simulink model "EKF"  (R2021a)
settings: Solver=VariableStepAuto  StartTime=0.0  StopTime=10.0  RelTol=1e-3
settings Model: Creator=migue  LastModifiedBy=migue

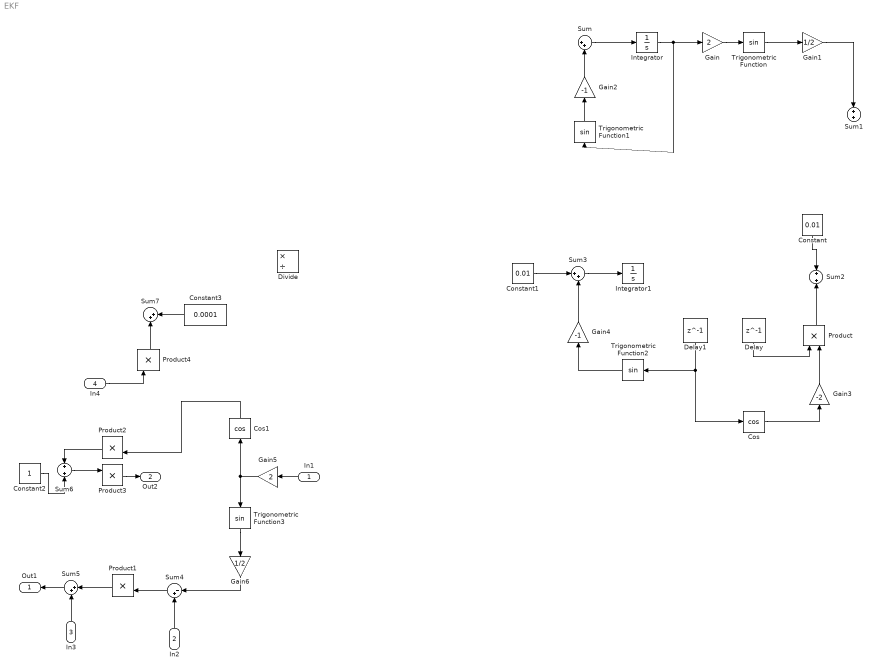
== system EKF ==
  In1 : Inport
  In2 : Inport  Port=2
  In3 : Inport  Port=3
  In4 : Inport  Port=4
  Constant : Constant  Value=0.01
  Constant1 : Constant  Value=0.01
  Constant2 : Constant
  Constant3 : Constant  Value=0.0001
  Cos : Trigonometry  Operator=cos
  Cos1 : Trigonometry  Operator=cos
  Delay : Delay  DelayLength=1  InitialCondition=0
  Delay1 : Delay  DelayLength=1  InitialCondition=0
  Divide : Product  Inputs=*/
  Gain : Gain  Gain=2
  Gain1 : Gain  Gain=1/2
  Gain2 : Gain  Gain=-1
  Gain3 : Gain  Gain=-2
  Gain4 : Gain  Gain=-1
  Gain5 : Gain  Gain=2
  Gain6 : Gain  Gain=1/2
  Integrator : Integrator
  Integrator1 : Integrator
  Product{,1..4} (5 alike) : Product
  Sum{,3,5,7} (4 alike) : Sum  Inputs=|++
  Sum1 : Sum  Inputs=+|+
  Sum2 : Sum
  Sum4 : Sum  Inputs=|-+
  Sum6 : Sum
  Trigonometric Function{,1..3} (4 alike) : Trigonometry
  Out1 : Outport
  Out2 : Outport  Port=2
  wires:
  Sum/1 -> Integrator/1
  Integrator/1 -> Gain/1, Trigonometric Function1/1
  Gain/1 -> Trigonometric Function/1
  Trigonometric Function/1 -> Gain1/1
  Gain1/1 -> Sum1/1
  Gain2/1 -> Sum/2
  Trigonometric Function1/1 -> Gain2/1
  Constant1/1 -> Sum3/1
  Sum3/1 -> Integrator1/1
  Gain4/1 -> Sum3/2
  Trigonometric Function2/1 -> Gain4/1
  Constant/1 -> Sum2/1
  Product/1 -> Sum2/2
  Gain3/1 -> Product/2
  Cos/1 -> Gain3/1
  Delay/1 -> Product/1
  Delay1/1 -> Cos/1, Trigonometric Function2/1
  Gain5/1 -> Cos1/1, Trigonometric Function3/1
  Trigonometric Function3/1 -> Gain6/1
  Gain6/1 -> Sum4/1
  In1/1 -> Gain5/1
  In2/1 -> Sum4/2
  Sum4/1 -> Product1/2
  Product1/1 -> Sum5/1
  In3/1 -> Sum5/2
  Sum5/1 -> Out1/1
  Cos1/1 -> Product2/2
  Product2/1 -> Sum6/1
  Sum6/1 -> Product3/1
  Product3/1 -> Out2/1
  Constant2/1 -> Sum6/2
  In4/1 -> Product4/1
  Product4/1 -> Sum7/1
  Constant3/1 -> Sum7/2
